simulink library "pathPosition_ul"  (R2018a)
settings: Solver=VariableStepAuto  StartTime=0.0  StopTime=10.0  RelTol=1e-3
values from neighbouring files (symbols this model uses):
  pathHeight_m = 10    [pathPosition_init.m]
  pathWidth_m = 50    [pathPosition_init.m]
settings Model: Creator=mcobb  LastModifiedBy=mcobb

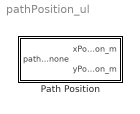
== system pathPosition_ul ==
  Path Position : Subsystem

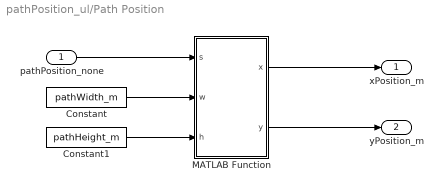
== system pathPosition_ul/Path Position ==
  pathPosition_none : Inport
  Constant : Constant  Value=pathWidth_m
  Constant1 : Constant  Value=pathHeight_m
  MATLAB Function : MATLAB Function  TreatAsAtomicUnit=on
  xPosition_m : Outport
  yPosition_m : Outport  Port=2
  wires:
  Constant1/1 -> MATLAB Function/3(h)
  pathPosition_none/1 -> MATLAB Function/1(s)
  Constant/1 -> MATLAB Function/2(w)
  MATLAB Function/1(x) -> xPosition_m/1
  MATLAB Function/2(y) -> yPosition_m/1

== matlab function pathPosition_ul/Path Position/MATLAB Function ==
  data: x output; s input; y output; w input; h input
function [x,y] = fcn(s,w,h)
p = pathPosition(s,w,h);
x = p(:,1);
y = p(:,2);
